simulink model "simulinkfile_project2_ME19B087"  (R2021a)
settings: Solver=VariableStepAuto  StartTime=0.0  StopTime=5.0  RelTol=1e-3
model workspace (MAT data in the model file):
  a1 = 238.4335
  a2 = 48422
  a3 = 2487100
  b0 = 0
  b1 = 117.5424
  b2 = 37259
  dc = 2.6815
libraries: simulink x1
settings Model: Creator=Benny  LastModifiedBy=Benny
settings SolverCC: ZeroCrossAlgorithm=Adaptive
settings DebuggingCC: IgnoredZcDiagnostic=none

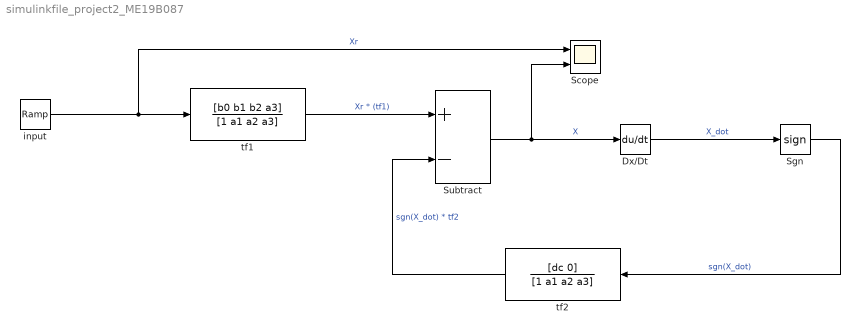
== system simulinkfile_project2_ME19B087 ==
  Dx/Dt : Derivative
  Scope : Scope  NumInputPorts=2
  Sgn : Signum
  Subtract : Sum  Inputs=+-
  input : simulink/Sources/Ramp  slope=1  start=0  InitialOutput=0
  tf1 : TransferFcn  Numerator=[b0 b1 b2 a3]  Denominator=[1 a1 a2 a3]
  tf2 : TransferFcn  Numerator=[dc 0]  Denominator=[1 a1 a2 a3]
  wires:
  input/1 -> Scope/1, tf1/1  "Xr"
  tf1/1 -> Subtract/1  "Xr * (tf1)"
  Subtract/1 -> Scope/2, Dx/Dt/1  "X"
  Dx/Dt/1 -> Sgn/1  "X_dot"
  Sgn/1 -> tf2/1  "sgn(X_dot)"
  tf2/1 -> Subtract/2  "sgn(X_dot) * tf2"
